simulink model "gm_sampleModel1911_3_sub"  (R2023a)
settings: Solver=VariableStepAuto  StartTime=0.0  StopTime=10.0  RelTol=1e-3
libraries: simulink x2
settings Model: Creator=user1  LastModifiedBy=user1
settings OptimizationCC: BlockReduction=off  ConditionallyExecuteInputs=off
settings DebuggingCC: InheritedTsInSrcMsg=none

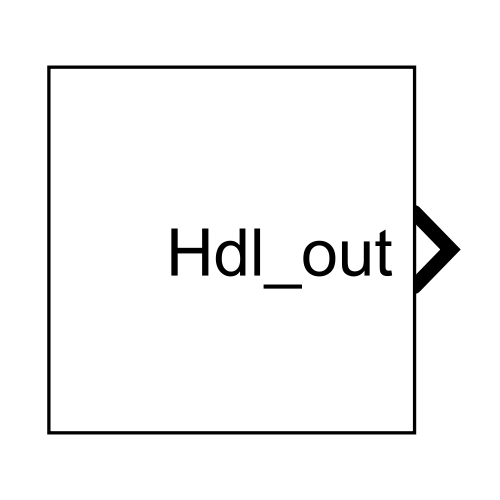
[thumbnail: Simulink's stored preview of the top-level diagram]
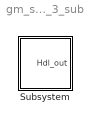
== system gm_sampleModel1911_3_sub ==
  Subsystem : Subsystem

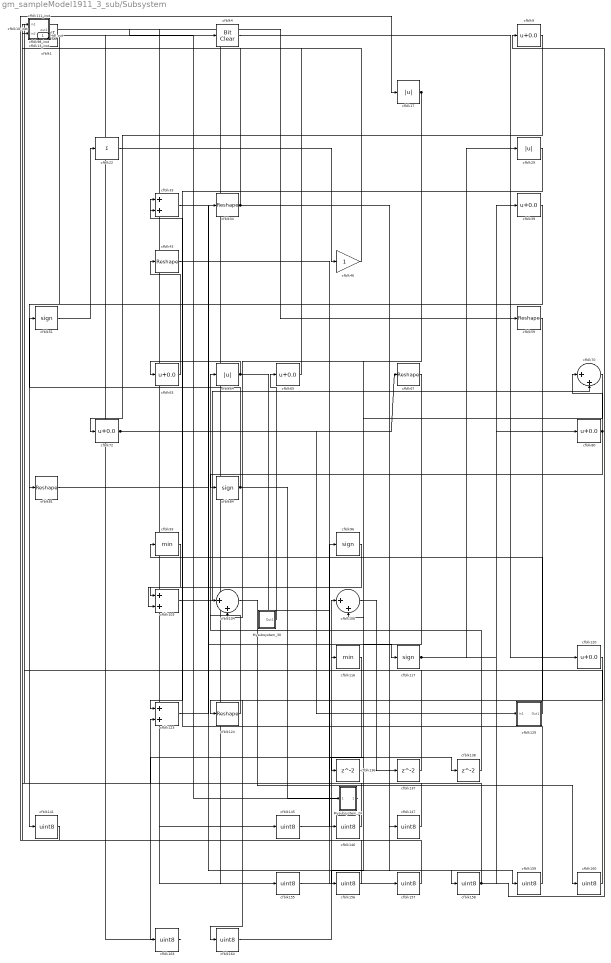
== system gm_sampleModel1911_3_sub/Subsystem ==
  Mysubsystem_24 : Subsystem
  Mysubsystem_30 : Subsystem
  cfblk1 : simulink/Logic and Bit Operations/Detect Increase  vinit=0.0  OutDataTypeStr=uint8
      settings: LibrarySourceBlock=|
      | hdlsllib/Logic and Bit
      | Operations/Detect
      | Increase
  cfblk103 : Sum  OutDataTypeStr=uint8
  cfblk104 : Sum  Inputs=|++  OutDataTypeStr=uint8
  cfblk106 : Sum  Inputs=|++  OutDataTypeStr=uint8
  cfblk10_inst : Subsystem
  cfblk111_inst : Subsystem
  cfblk116 : MinMax  OutDataTypeStr=uint8
  cfblk{51,84,96,117} (4 alike) : Signum
  cfblk{9,39,63,65,72,80,120} (7 alike) : Bias  Bias=0.0  SaturateOnIntegerOverflow=off
  cfblk123 : Sum  OutDataTypeStr=uint8
  cfblk{34,43,59,67,81,124} (6 alike) : Reshape
  cfblk129 : Subsystem
  cfblk136 : Delay  SampleTime=1
  cfblk137 : Delay  SampleTime=1
  cfblk138 : Delay  SampleTime=1
  cfblk13_inst : Subsystem
  cfblk{141,145..147,155..160,163..164} (12 alike) : DataTypeConversion  OutDataTypeStr=uint8  SaturateOnIntegerOverflow=off  RndMeth=Floor
  cfblk17 : Abs  OutDataTypeStr=uint8  SaturateOnIntegerOverflow=off
  cfblk22 : Sum  Inputs=+  OutDataTypeStr=uint8
  cfblk29 : Abs  OutDataTypeStr=uint8  SaturateOnIntegerOverflow=off
  cfblk33 : Sum  OutDataTypeStr=uint8
  cfblk4 : simulink/Logic and Bit Operations/Bit Clear  iBit=0
      settings: LibrarySourceBlock=|
      | hdlsllib/Logic and Bit
      | Operations/Bit Clear
  cfblk46 : Gain  OutDataTypeStr=uint8
  cfblk64 : Abs  OutDataTypeStr=uint8  SaturateOnIntegerOverflow=off
  cfblk70 : Sum  Inputs=|++  OutDataTypeStr=uint8
  cfblk93 : MinMax  OutDataTypeStr=uint8
  cfblk98_inst : Subsystem
  Hdl_out : Outport  OutDataTypeStr=uint8  SampleTime=1
  wires:
  Mysubsystem_24/1(Out1) -> cfblk1/1
  Mysubsystem_30/1(Out1) -> cfblk65/1
  cfblk1/1 -> cfblk141/1
  cfblk10_inst/1(out1) -> cfblk155/1
  cfblk103/1 -> cfblk70/2
  cfblk104/1 -> cfblk160/1
  cfblk106/1 -> cfblk137/1
  cfblk111_inst/1(out1) -> cfblk59/1, cfblk157/1
  cfblk116/1 -> cfblk163/1
  cfblk117/1 -> cfblk80/1, cfblk29/1
  cfblk120/1 -> cfblk124/1
  cfblk123/1 -> cfblk34/1
  cfblk124/1 -> cfblk64/1
  cfblk129/1(Out1) -> cfblk93/1
  cfblk13_inst/1(out1) -> cfblk145/1
  cfblk136/1 -> cfblk159/1
  cfblk137/1 -> cfblk98_inst/1(in1)
  cfblk138/1 -> cfblk104/1
  cfblk141/1 -> cfblk17/1
  cfblk145/1 -> cfblk106/1
  cfblk146/1 -> cfblk13_inst/1(in1)
  cfblk147/1 -> cfblk13_inst/2(in2)
  cfblk155/1 -> cfblk96/1
  cfblk156/1 -> cfblk10_inst/1(in1)
  cfblk157/1 -> cfblk10_inst/2(in2)
  cfblk158/1 -> cfblk9/1, cfblk39/1, cfblk123/2
  cfblk159/1 -> cfblk33/1
  cfblk160/1 -> cfblk33/2
  cfblk163/1 -> Hdl_out/1
  cfblk164/1 -> cfblk116/1
  cfblk17/1 -> cfblk106/2, cfblk104/2
  cfblk22/1 -> cfblk46/1
  cfblk29/1 -> cfblk103/1
  cfblk33/1 -> cfblk158/1
  cfblk34/1 -> cfblk98_inst/2(in2), cfblk147/1
  cfblk39/1 -> cfblk81/1
  cfblk4/1 -> cfblk120/1
  cfblk43/1 -> cfblk138/1
  cfblk46/1 -> cfblk111_inst/1(in1)
  cfblk51/1 -> cfblk22/1
  cfblk59/1 -> cfblk164/1
  cfblk63/1 -> cfblk43/1
  cfblk64/1 -> cfblk63/1, cfblk146/1
  cfblk65/1 -> cfblk111_inst/2(in2)
  cfblk67/1 -> cfblk136/1
  cfblk70/1 -> cfblk156/1
  cfblk72/1 -> cfblk67/1, cfblk129/1(In1)
  cfblk80/1 -> cfblk84/1, cfblk70/1
  cfblk81/1 -> cfblk117/1
  cfblk84/1 -> cfblk51/1, Mysubsystem_24/1(In1)
  cfblk9/1 -> cfblk72/1
  cfblk93/1 -> cfblk103/2
  cfblk96/1 -> cfblk123/1
  cfblk98_inst/1(out1) -> cfblk4/1

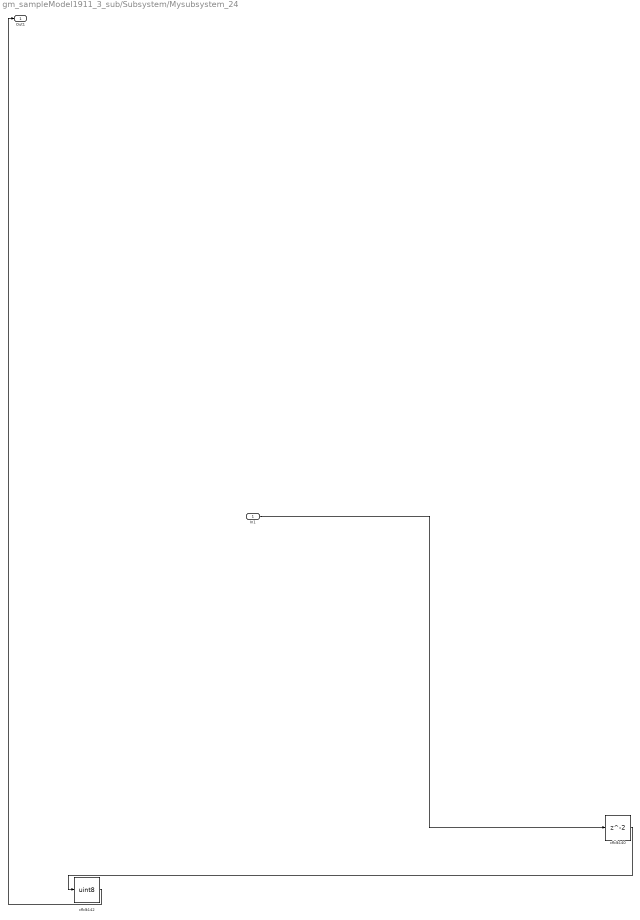
== system gm_sampleModel1911_3_sub/Subsystem/Mysubsystem_24 ==
  In1 : Inport  OutDataTypeStr=uint8  PortDimensions=1  SampleTime=1
  cfblk140 : Delay  SampleTime=1
  cfblk142 : DataTypeConversion  OutDataTypeStr=uint8  SaturateOnIntegerOverflow=off  RndMeth=Floor
  Out1 : Outport  SampleTime=1
  wires:
  In1/1 -> cfblk140/1
  cfblk140/1 -> cfblk142/1
  cfblk142/1 -> Out1/1

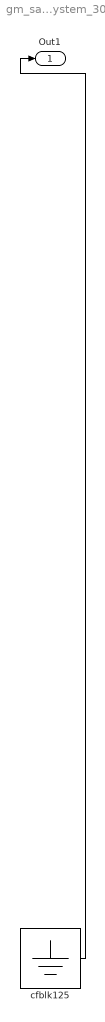
== system gm_sampleModel1911_3_sub/Subsystem/Mysubsystem_30 ==
  cfblk125 : Ground
  Out1 : Outport  SampleTime=1
  wires:
  cfblk125/1 -> Out1/1

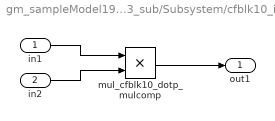
== system gm_sampleModel1911_3_sub/Subsystem/cfblk10_inst ==
  in1 : Inport  OutDataTypeStr=uint8  SampleTime=1
  in2 : Inport  Port=2  OutDataTypeStr=uint8  SampleTime=1
  mul_cfblk10_dotp_mulcomp : Product  Inputs=**  OutDataTypeStr=uint8  SampleTime=1
  out1 : Outport  OutDataTypeStr=uint8  SampleTime=1
  wires:
  in1/1 -> mul_cfblk10_dotp_mulcomp/1
  in2/1 -> mul_cfblk10_dotp_mulcomp/2
  mul_cfblk10_dotp_mulcomp/1 -> out1/1

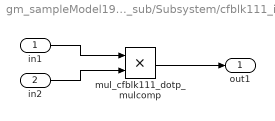
== system gm_sampleModel1911_3_sub/Subsystem/cfblk111_inst ==
  in1 : Inport  OutDataTypeStr=uint8  SampleTime=1
  in2 : Inport  Port=2  OutDataTypeStr=uint8  SampleTime=1
  mul_cfblk111_dotp_mulcomp : Product  Inputs=**  OutDataTypeStr=uint8  SampleTime=1
  out1 : Outport  OutDataTypeStr=uint8  SampleTime=1
  wires:
  in1/1 -> mul_cfblk111_dotp_mulcomp/1
  in2/1 -> mul_cfblk111_dotp_mulcomp/2
  mul_cfblk111_dotp_mulcomp/1 -> out1/1

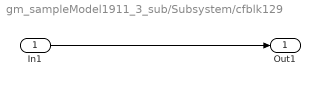
== system gm_sampleModel1911_3_sub/Subsystem/cfblk129 ==
  In1 : Inport  OutDataTypeStr=uint8  PortDimensions=1  SampleTime=1
  Out1 : Outport  SampleTime=1
  wires:
  In1/1 -> Out1/1

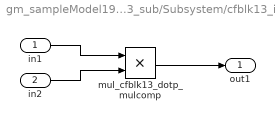
== system gm_sampleModel1911_3_sub/Subsystem/cfblk13_inst ==
  in1 : Inport  OutDataTypeStr=uint8  SampleTime=1
  in2 : Inport  Port=2  OutDataTypeStr=uint8  SampleTime=1
  mul_cfblk13_dotp_mulcomp : Product  Inputs=**  OutDataTypeStr=uint8  SampleTime=1
  out1 : Outport  OutDataTypeStr=uint8  SampleTime=1
  wires:
  in1/1 -> mul_cfblk13_dotp_mulcomp/1
  in2/1 -> mul_cfblk13_dotp_mulcomp/2
  mul_cfblk13_dotp_mulcomp/1 -> out1/1

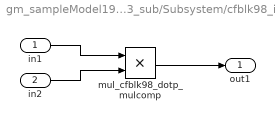
== system gm_sampleModel1911_3_sub/Subsystem/cfblk98_inst ==
  in1 : Inport  OutDataTypeStr=uint8  SampleTime=1
  in2 : Inport  Port=2  OutDataTypeStr=uint8  SampleTime=1
  mul_cfblk98_dotp_mulcomp : Product  Inputs=**  OutDataTypeStr=uint8  SampleTime=1
  out1 : Outport  OutDataTypeStr=uint8  SampleTime=1
  wires:
  in1/1 -> mul_cfblk98_dotp_mulcomp/1
  in2/1 -> mul_cfblk98_dotp_mulcomp/2
  mul_cfblk98_dotp_mulcomp/1 -> out1/1
